simulink model "simulacao_continuo"  (R2021b)
settings: Solver=VariableStepAuto  StartTime=0.0  StopTime=5  RelTol=1e-3
values from neighbouring files (symbols this model uses):
  A = [0, 0, 1, 0 ... (first row only)    [ganhos_lqr_continuo.m]    (also in ganhos_lqr_discreto.m)
  B = [0 ... (first row only)    [ganhos_lqr_continuo.m]    (also in ganhos_lqr_discreto.m)
  C = eye(4)    [ganhos_lqr_continuo.m]    (also in ganhos_lqr_discreto.m)
  D = [0;0;0;0]    [ganhos_lqr_continuo.m]    (also in ganhos_lqr_discreto.m)
undefined symbols (not defined in the file or in its folder): K
settings Model: Creator=marco  LastModifiedBy=marco
settings SolverCC: AlgebraicLoopSolver=TrustRegion

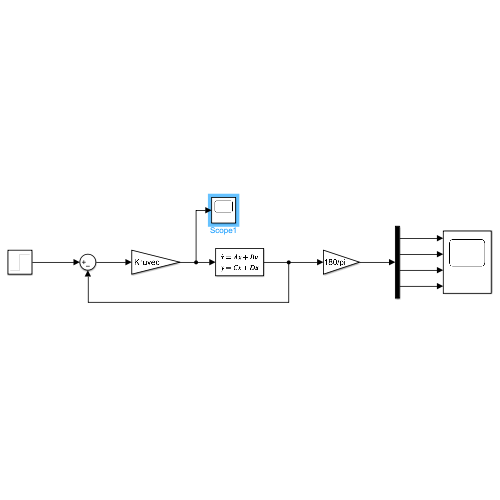
[thumbnail: Simulink's stored preview of the top-level diagram]
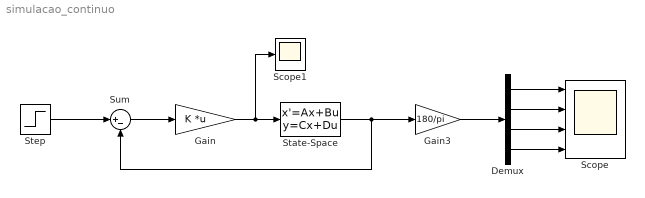
== system simulacao_continuo ==
  Demux : Demux
  Gain : Gain  Gain=K  Multiplication=Matrix(K*u) (u vector)
  Gain3 : Gain  Gain=180/pi
  Scope : Scope  NumInputPorts=4
  Scope1 : Scope
  State-Space : StateSpace  A=A  B=B  C=C  D=D  InitialCondition=[0,5*pi/180,0,0]
  Step : Step  Time=0  After=0  SampleTime=0
  Sum : Sum  Inputs=|+-
  wires:
  Gain/1 -> Scope1/1, State-Space/1
  Step/1 -> Sum/1
  Sum/1 -> Gain/1
  Demux/3 -> Scope/3
  Demux/4 -> Scope/4
  State-Space/1 -> Sum/2, Gain3/1
  Demux/1 -> Scope/1
  Demux/2 -> Scope/2
  Gain3/1 -> Demux/1
